simulink model "Exp3_Simulink2"  (R2018b)
settings: Solver=VariableStepAuto  StartTime=0.0  StopTime=10.0  RelTol=1e-3
undefined symbols (not defined in the file or in its folder): Q, QuaternionMul, R
settings Model: Creator=Administrator  LastModifiedBy=Administrator

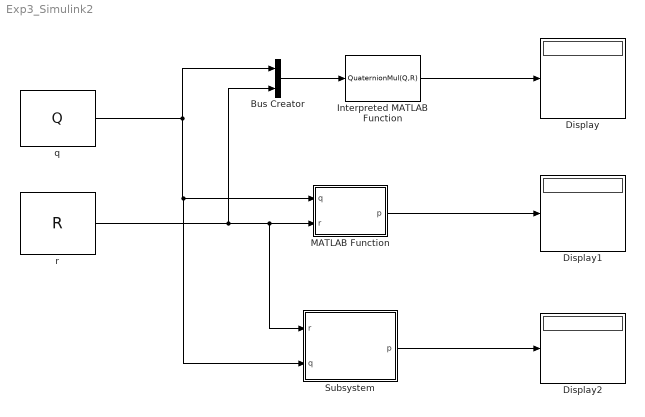
== system Exp3_Simulink2 ==
  Bus Creator : BusCreator  Inputs=2
  Display : Display
  Display1 : Display
  Display2 : Display
  Interpreted MATLAB Function : MATLABFcn  MATLABFcn=QuaternionMul(Q,R)
  MATLAB Function : MATLAB Function  TreatAsAtomicUnit=on
  Subsystem : Subsystem
  q : Constant  Value=Q
  r : Constant  Value=R
  wires:
  Interpreted MATLAB Function/1 -> Display/1
  MATLAB Function/1(p) -> Display1/1
  Subsystem/1(p) -> Display2/1
  r/1 -> Bus Creator/2, Subsystem/1(r), MATLAB Function/2(r)
  q/1 -> Bus Creator/1, Subsystem/2(q), MATLAB Function/1(q)
  Bus Creator/1 -> Interpreted MATLAB Function/1

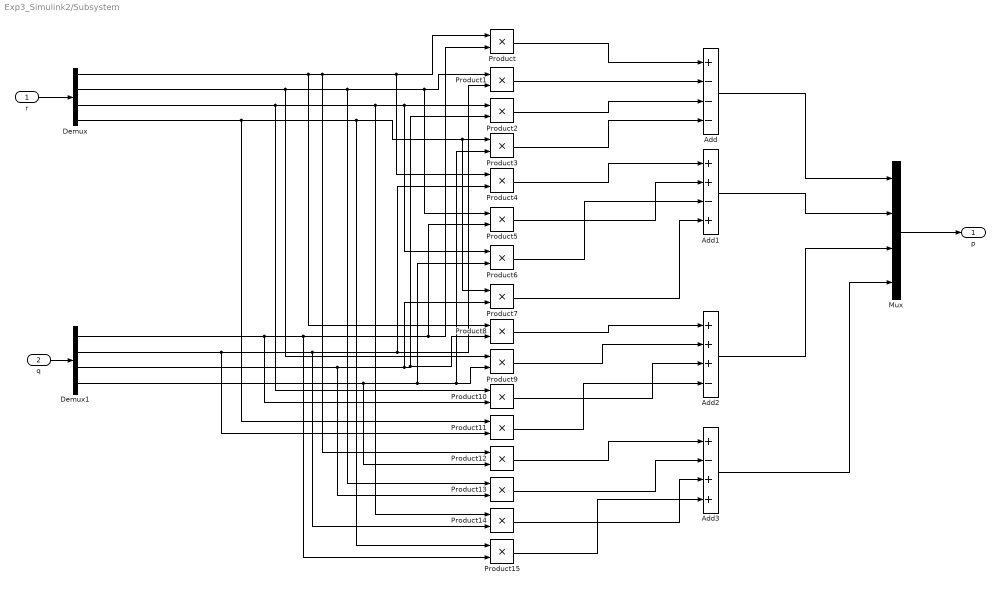
== system Exp3_Simulink2/Subsystem ==
  r : Inport
  q : Inport  Port=2
  Add : Sum  Inputs=+---
  Add1 : Sum  Inputs=++-+
  Add2 : Sum  Inputs=+++-
  Add3 : Sum  Inputs=+-++
  Demux : Demux
  Demux1 : Demux
  Mux : Mux
  Product{,1..15} (16 alike) : Product
  p : Outport
  wires:
  r/1 -> Demux/1
  q/1 -> Demux1/1
  Mux/1 -> p/1
  Demux/1 -> Product8/1, Product12/1, Product4/1, Product/1
  Demux1/1 -> Product10/2, Product15/2, Product5/2, Product/2
  Product/1 -> Add/1
  Demux/2 -> Product9/1, Product13/1, Product5/1, Product1/1
  Demux1/2 -> Product11/2, Product14/2, Product4/2, Product1/2
  Product1/1 -> Add/2
  Demux/3 -> Product10/1, Product14/1, Product6/1, Product2/1
  Demux1/3 -> Product13/2, Product7/2, Product8/2, Product2/2
  Demux1/4 -> Product12/2, Product9/2, Product3/2, Product6/2
  Product2/1 -> Add/3
  Product3/1 -> Add/4
  Add/1 -> Mux/1
  Product4/1 -> Add1/1
  Product5/1 -> Add1/2
  Product6/1 -> Add1/3
  Product7/1 -> Add1/4
  Add1/1 -> Mux/2
  Product8/1 -> Add2/1
  Product9/1 -> Add2/2
  Product10/1 -> Add2/3
  Product11/1 -> Add2/4
  Product12/1 -> Add3/1
  Product13/1 -> Add3/2
  Product14/1 -> Add3/3
  Product15/1 -> Add3/4
  Add2/1 -> Mux/3
  Add3/1 -> Mux/4
  Demux/4 -> Product11/1, Product15/1, Product7/1, Product3/1

== matlab function Exp3_Simulink2/MATLAB Function ==
  data: q input; p output; r input
function p = fcn(q,r)

p = [r(1)*q(1)-r(2)*q(2)-r(3)*q(3)-r(4)*q(4)
    r(1)*q(2)+r(2)*q(1)-r(3)*q(4)+r(4)*q(3)
    r(1)*q(3)+r(2)*q(4)+r(3)*q(1)-r(4)*q(2)
    r(1)*q(4)-r(2)*q(3)+r(3)*q(2)+r(4)*q(1)]';
